simulink model "test_stage_2"  (R2020b)
settings: Solver=FixedStepAuto  StartTime=0.0  StopTime=0.4  FixedStep=0.001  RelTol=1e-3
values from neighbouring files (symbols this model uses):
  a_max = F_max / m_R    (= 10)    [multi_stage_safety_aware_setup.m]    (also in stage_II_subsystem.m = 3)
  b0 = 20    [FSM.m]    (also in multi_stage_safety_aware_setup.m = 2 * sqrt(m_R * k0))
  j_max = 300    [multi_stage_safety_aware_setup.m]    (also in stage_II_subsystem.m = 30)
  k0 = 100    [FSM.m]    (also in multi_stage_safety_aware_setup.m)
  m_R = 1    [multi_stage_safety_aware_setup.m]    (also in stage_II_subsystem.m)
  T_R = 0.001    [multi_stage_safety_aware_setup.m]    (also in stage_II_subsystem.m)
  v0 = obj.v0    [braking_memory_rapid.m]    (also in braking_memory_trapezoid.m; multi_stage_safety_aware_setup.m = 1)
settings Model: PauseTimes=0.1  Creator=kika  LastModifiedBy=kika

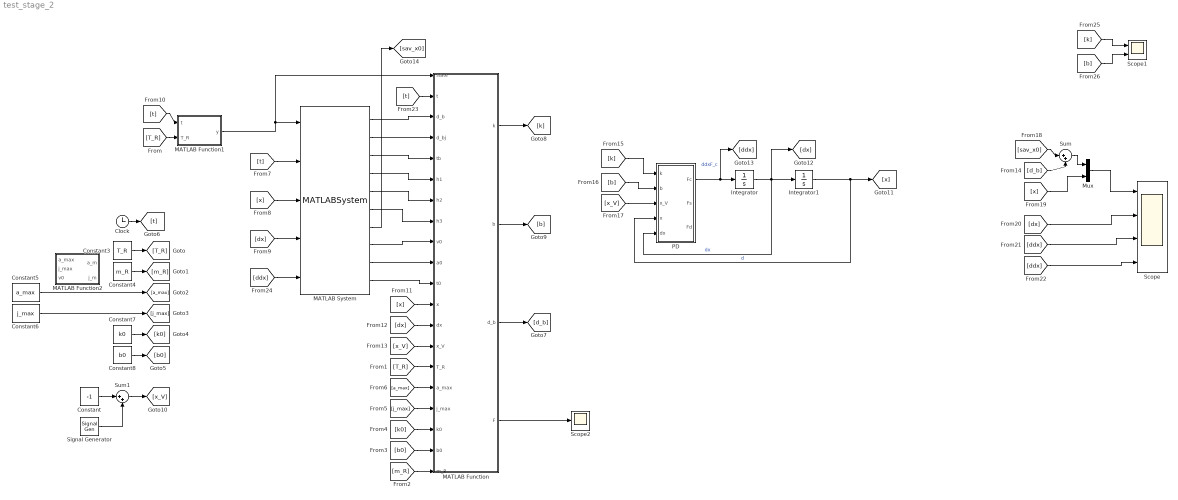
== system test_stage_2 ==
  Clock : Clock
  Constant : Constant  Value=-1
  Constant3 : Constant  Value=T_R
  Constant4 : Constant  Value=m_R
  Constant5 : Constant  Value=a_max
  Constant6 : Constant  Value=j_max
  Constant7 : Constant  Value=k0
  Constant8 : Constant  Value=b0
  Integrator : Integrator  InitialCondition=v0
  Integrator1 : Integrator
  MATLAB Function : MATLAB Function  TreatAsAtomicUnit=on
  MATLAB Function1 : MATLAB Function  TreatAsAtomicUnit=on
  MATLAB Function2 : MATLAB Function  TreatAsAtomicUnit=on
  MATLAB System : MATLABSystem  System=braking_memory  a_max=a_max  j_max=j_max  T_R=T_R  x0_=x0  v0_=v0  x_V0=x_V0  k0=k0  b0=b0  SimulateUsing=Code generation
      mask Type: braking_memory
      mask Display:
      | disp('braking_memory');
      | port_label('input',1,'state');
      | port_label('input',2,'t');
      | port_label('input',3,'x');
      | port_label('input',4,'dx');
      | port_label('input',5,'ddx');
      | port_label('output',1,'d_b0');
      | port_label('output',2,'d_b_j0');
      | port_label('output',3,'t_b0');
      | port_label('output',4,'h10');
      | port_label('output',5,'h20');
      | port_label('output',6,'h30');
      | port_label('output',7,'x0');
      | port_label('output',8,'v0');
      | port_label('output',9,'a0');
      | port_label('output',10,'t0');
  Mux : Mux  Inputs=2
  PD : MATLAB Function  TreatAsAtomicUnit=on
  Scope : Scope  NumInputPorts=4
  Scope1 : Scope  NumInputPorts=2
  Scope2 : Scope
  Signal Generator : SignalGenerator  Frequency=0.3  Units=rad/sec
  Sum : Sum  Inputs=|++
  Sum1 : Sum  Inputs=|++
  wires:
  PD/1(Fc) -> [ddx], Integrator/1  "ddxF_c"
  Integrator/1 -> [dx], PD/5(dx), Integrator1/1  "dx"
  Integrator1/1 -> [x], PD/4(x)  "d"
  [x_V] -> PD/3(x_V)
  Mux/1 -> Scope/1
  MATLAB Function1/1(y) -> MATLAB Function/1(state), MATLAB System/1
  Constant3/1 -> [T_R]
  Constant4/1 -> [m_R]
  Constant6/1 -> [j_max]
  Constant7/1 -> [k0]
  Constant8/1 -> [b0]
  [T_R] -> MATLAB Function1/2(T_R)
  [T_R] -> MATLAB Function/15(T_R)
  [m_R] -> MATLAB Function/20(m_R)
  [b0] -> MATLAB Function/19(b0)
  [k0] -> MATLAB Function/18(k0)
  [j_max] -> MATLAB Function/17(j_max)
  [a_max] -> MATLAB Function/16(a_max)
  Constant5/1 -> [a_max]
  Sum/1 -> Mux/1
  [t] -> MATLAB System/2
  [x] -> MATLAB System/3
  [dx] -> MATLAB System/4
  [ddx] -> MATLAB System/5
  [t] -> MATLAB Function1/1(t)
  Clock/1 -> [t]
  [x] -> MATLAB Function/12(x)
  [dx] -> MATLAB Function/13(dx)
  [x_V] -> MATLAB Function/14(x_V)
  MATLAB Function/3(d_b) -> [d_b]
  [d_b] -> Sum/2
  MATLAB Function/1(k) -> [k]
  MATLAB Function/2(b) -> [b]
  [k] -> PD/1(k)
  [b] -> PD/2(b)
  Constant/1 -> Sum1/1
  [sav_x0] -> Sum/1
  [x] -> Mux/2
  [dx] -> Scope/2
  [ddx] -> Scope/3
  [ddx] -> Scope/4
  [t] -> MATLAB Function/2(t)
  Sum1/1 -> [x_V]
  Signal Generator/1 -> Sum1/2
  [k] -> Scope1/1
  [b] -> Scope1/2
  MATLAB Function/4(F) -> Scope2/1
  MATLAB System/1 -> MATLAB Function/3("d_b ")
  MATLAB System/2 -> MATLAB Function/4(d_bj)
  MATLAB System/3 -> MATLAB Function/5(tb)
  MATLAB System/4 -> MATLAB Function/6(h1)
  MATLAB System/5 -> MATLAB Function/7(h2)
  MATLAB System/6 -> MATLAB Function/8(h3)
  MATLAB System/7 -> [sav_x0]
  MATLAB System/8 -> MATLAB Function/9(v0)
  MATLAB System/9 -> MATLAB Function/10(a0)
  MATLAB System/10 -> MATLAB Function/11(t0)

== matlab function test_stage_2/MATLAB Function1 ==
  data: t input; y output; T_R input
function y = fcn(t, T_R)
    y = 0;
    
    time_to_switch = 0.100;
    if t == time_to_switch
        y = 1;
    end
    if t > time_to_switch
        y = 2;
    end

== matlab function test_stage_2/MATLAB Function ==
  data: state input; t input; d_b input; d_bj input; tb input; h1 input; h2 input; h3 input; v0 input; a0 input; t0 input; x input; k output; b output; dx input; x_V input; d_b output; T_R input; a_max input; j_max input; k0 input; b0 input; m_R input; F output
function [k,b, d_b, F] = safety_SII(state, t, d_b, d_bj, tb, h1, h2, h3, v0, a0, t0, x, dx, x_V, T_R, a_max, j_max, k0, b0, m_R)
  
    k = k0;
    b = b0;
    
    F = 0;
    
    tk = t - t0;
    if state == 2
        kI = 0; 
        k = (kI-k0) * (tk / (tb)) + k0;   % tk <= tb
        if k < 0
            k = 0;
        end

        % rapid braking
%         F = 0;
%         if tk < h1
%             F = m_R * (a0 - j_max * tk);
%         elseif tk <= tb
%             F = -m_R * a_max;
%         end
%         
        % trapezoid
        F = 0;
        if tk < h1
            F = m_R * (a0 - j_max * tk);
        elseif tk <= h1 + h2
            F = -m_R * a_max;
        elseif tk < h1+h2+h3
            F = - m_R * (a_max + j_max * (h1+h2 - tk));
        end
        
        b = abs((k * (x_V - x) - F) / dx);
    end

== matlab function test_stage_2/PD ==
  data: k input; b input; x_V input; x input; Fc output; dx input; Fs output; Fd output
function [Fc, Fs, Fd]= PD(k, b, x_V, x, dx)

Fs = k * (x_V -x);
Fd = b * dx;
Fc = Fs - Fd;

== matlab function test_stage_2/MATLAB Function2 ==
  data: a_max input; a_m output; j_max input; v0 input; j_m output
function [a_m, j_m] = fcn(a_max, j_max, v0)

    a_m = sign(v0) * a_max;
    j_m = sign(v0) * j_max;
